simulink model "vekt_shim_PMSM"  (R2019b)
settings: Solver=ode4  StartTime=0.0  StopTime=10  FixedStep=1e-5  RelTol=1e-3
libraries: powerlib x4, simulink x3, powerlib_meascontrol x1
settings Model: Creator=Sozonov_AA  LastModifiedBy=Андрей
settings DataIOCC: SaveOutput=off  SaveTime=off
settings OptimizationCC: DefaultParameterBehavior=Inlined  InlineInvariantSignals=on  EnhancedBackFolding=on  PassReuseOutputArgsAs=Individual arguments  StateBitsets=on  DataBitsets=on  ZeroExternalMemoryAtStartup=off  ZeroInternalMemoryAtStartup=off  NoFixptDivByZeroProtection=on  EfficientFloat2IntCast=on  OptimizeBlockOrder=speed  DifferentSizesBufferReuse=on  EfficientTunableParamExpr=on
settings DebuggingCC: ParameterTunabilityLossMsg=error
settings SFSimCC: MATLABDynamicMemAlloc=off  CustomCodeUndefinedFunction=UseInterfaceOnly
settings RTWCC: SystemTargetFile=ert.tlc  TemplateMakefile=ert_default_tmf  GenerateReport=on  RTWVerbose=off  IncludeHyperlinkInReport=on  LaunchReport=on  GenerateTraceInfo=on  GenerateTraceReport=on  GenerateTraceReportSl=on  GenerateTraceReportSf=on  GenerateTraceReportEml=on
settings CodeAppCC: ForceParamTrailComments=on  IgnoreCustomStorageClasses=off  OperatorAnnotations=on  SimulinkDataObjDesc=on  SFDataObjDesc=on  CustomSymbolStrGlobalVar=rt$N$M  CustomSymbolStrType=$N$M  CustomSymbolStrFcn=$N$M$F  CustomSymbolStrMacro=$N$M  InsertBlockDesc=on
settings ERTTargetCC: TargetLangStandard=C99 (ISO)  GenerateSampleERTMain=on  IncludeMdlTerminateFcn=off  CombineSignalStateStructs=on  PurelyIntegerCode=on  SupportNonFinite=off  InlinedParameterPlacement=NonHierarchical  ERTCustomFileTemplate=example_file_process.tlc

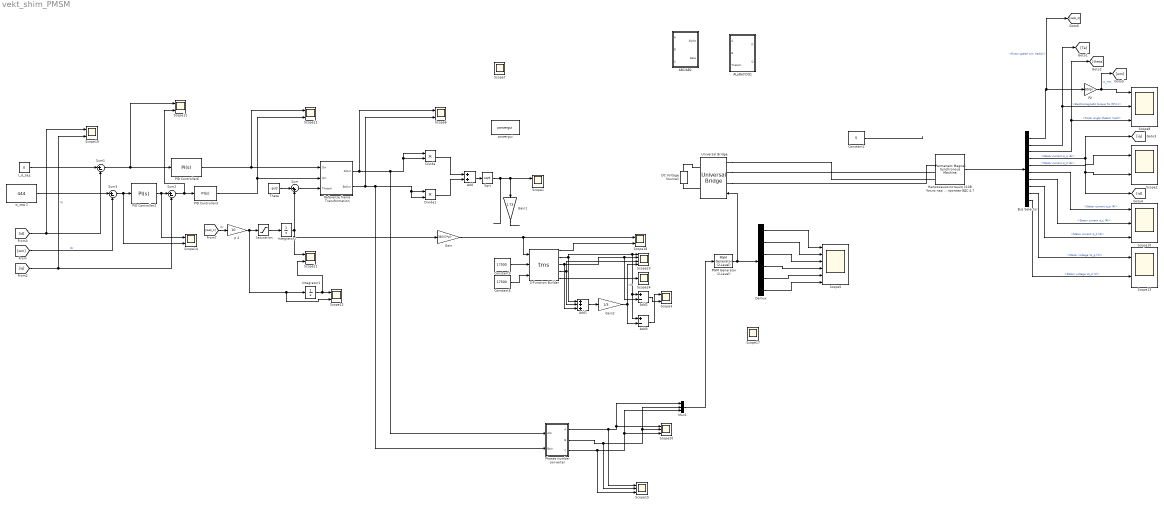
== system vekt_shim_PMSM ==
  "\tReferense frame Transformation" : Subsystem
  ABC/AB2 : Subsystem
  ALpBet\DQ1 : Subsystem
  Add : Sum
  Add1 : Sum  Inputs=+++
  Add2 : Sum  Inputs=+-
  Add3 : Sum  Inputs=+-
  Bus Selector : BusSelector  OutputSignals=Rotor speed wm (rad/s),Electromagnetic torque Te (N*m),Rotor angle thetam (rad),Stator current is_q (A),Stator current is_d (A),Stator current is_a (A),Stator current is_c (A),Stator current is_b (A),Stator voltage Vs_q (V),Stator voltage Vs_d (V)
  Constant2 : Constant  Value=5
  Constant3 : Constant  Value=17500
  Constant5 : Constant  Value=17500
  DC Voltage Source1 : powerlib/Electrical Sources/DC Voltage Source  Amplitude=310  Measurements=None
      settings: SourceProductName=Simscape Electrical
  Demux : Demux  Outputs=6
  Divide : Product  Inputs=**
  Divide1 : Product  Inputs=**
  Gain : Gain  Gain=360/(2*pi)
  Gain1 : Gain  Gain=1.73
  Gain2 : Gain  Gain=1/3
  I_d_зад : Constant  Value=0
  Integrator1 : Integrator  UpperSaturationLimit=2*pi  LowerSaturationLimit=0  WrappedStateUpperValue=2*pi  WrappedStateLowerValue=0  ZeroCross=off
  Integrator2 : Integrator  UpperSaturationLimit=2*pi  LowerSaturationLimit=0  WrapState=on  WrappedStateUpperValue=2*pi  WrappedStateLowerValue=0  ZeroCross=off
  Mux1 : Mux  Inputs=3
  P2 : Gain  Gain=30/pi
  PID Controller2 : simulink/Continuous/PID Controller  Controller=PI  Form=Ideal  TimeDomain=Continuous-time  SampleTime=-1  IntegratorMethod=Forward Euler  FilterMethod=Forward Euler  ControllerParametersSource=internal  P=16/444  I=(16/444)*150  D=0  UseFilter=on  N=100  TunerSelectOption=Transfer Function Based (PID Tuner App)  InitialConditionSource=internal  InitialConditionForIntegrator=0  InitialConditionForFilter=0  DifferentiatorICPrevScaledInput=0  ExternalReset=none  TrackingMode=off  Kt=1  LimitOutput=on  UpperSaturationLimit=1000  LowerSaturationLimit=-1000  LinearizeAsGain=on  AntiWindupMode=none  Kb=1  POutMin=[]  POutMax=[]  IOutMin=[]  IOutMax=[]  DOutMin=[]  DOutMax=[]  NOutMin=[]  NOutMax=[]  SumOutMin=[]  SumOutMax=[]  SaturationOutMin=[]  SaturationOutMax=[]  PParamMin=[]  PParamMax=[]  IParamMin=[]  IParamMax=[]  DParamMin=[]  DParamMax=[]  NParamMin=[]  NParamMax=[]  KbParamMin=[]  KbParamMax=[]  KtParamMin=[]  KtParamMax=[]  KbOutMin=[]  KbOutMax=[]  KtOutMin=[]  KtOutMax=[]  IntegratorOutMin=[]  IntegratorOutMax=[]  FilterOutMin=[]  FilterOutMax=[]  SumI1OutMin=[]  SumI1OutMax=[]  SumI2OutMin=[]  SumI2OutMax=[]  SumI3OutMin=[]  SumI3OutMax=[]  SumI4OutMin=[]  SumI4OutMax=[]  SumDOutMin=[]  SumDOutMax=[]  DifferentiatorOutMin=[]  DifferentiatorOutMax=[]  FilterDiffOutCoefMin=[]  FilterDiffOutCoefMax=[]  ReciprocalOutMin=[]  ReciprocalOutMax=[]  SumDenOutMin=[]  SumDenOutMax=[]  SumNumOutMin=[]  SumNumOutMax=[]  DivideOutMin=[]  DivideOutMax=[]  IntegratorContinuousStateAttributes=''  IntegratorStateMustResolveToSignalObject=off  IntegratorRTWStateStorageClass=Auto  FilterContinuousStateAttributes=''  FilterStateMustResolveToSignalObject=off  FilterRTWStateStorageClass=Auto  ParallelPVariant=Passthrough  IdealPVariant=InternalParameters  IVariant=InternalParameters  DVariant=Disabled  IntegratorVariant=Continuous  SatVariant=Enabled  AWVariant=Passthrough  PCopyVariant=Disabled  TRVariant=Disabled  FdbkBlocksVariant=Forward  IdealPFdbkVariant=Disabled  SatFdbkVariant=Disabled  DerivativeFilterVariant=Disabled  NVariant=Disabled  NCopyVariant=Disabled_SignalSpec  FilterICVariant=Disabled  IntegratorICVariant=InternalICs  ExternalResetVariant=Disabled  TRSumVariant=Passthrough  SumFdbkVariant=Disabled  SumVariant=Sum_PI
  PID Controller3 : simulink/Continuous/PID Controller  Controller=PI  Form=Ideal  TimeDomain=Continuous-time  SampleTime=-1  IntegratorMethod=Forward Euler  FilterMethod=Forward Euler  ControllerParametersSource=internal  P=220/0.5  I=(220/0.5)*4  D=0  UseFilter=on  N=100  TunerSelectOption=Transfer Function Based (PID Tuner App)  InitialConditionSource=internal  InitialConditionForIntegrator=0  InitialConditionForFilter=0  DifferentiatorICPrevScaledInput=0  ExternalReset=none  TrackingMode=off  Kt=1  LimitOutput=on  UpperSaturationLimit=1000  LowerSaturationLimit=-1000  LinearizeAsGain=on  AntiWindupMode=none  Kb=1  POutMin=[]  POutMax=[]  IOutMin=[]  IOutMax=[]  DOutMin=[]  DOutMax=[]  NOutMin=[]  NOutMax=[]  SumOutMin=[]  SumOutMax=[]  SaturationOutMin=[]  SaturationOutMax=[]  PParamMin=[]  PParamMax=[]  IParamMin=[]  IParamMax=[]  DParamMin=[]  DParamMax=[]  NParamMin=[]  NParamMax=[]  KbParamMin=[]  KbParamMax=[]  KtParamMin=[]  KtParamMax=[]  KbOutMin=[]  KbOutMax=[]  KtOutMin=[]  KtOutMax=[]  IntegratorOutMin=[]  IntegratorOutMax=[]  FilterOutMin=[]  FilterOutMax=[]  SumI1OutMin=[]  SumI1OutMax=[]  SumI2OutMin=[]  SumI2OutMax=[]  SumI3OutMin=[]  SumI3OutMax=[]  SumI4OutMin=[]  SumI4OutMax=[]  SumDOutMin=[]  SumDOutMax=[]  DifferentiatorOutMin=[]  DifferentiatorOutMax=[]  FilterDiffOutCoefMin=[]  FilterDiffOutCoefMax=[]  ReciprocalOutMin=[]  ReciprocalOutMax=[]  SumDenOutMin=[]  SumDenOutMax=[]  SumNumOutMin=[]  SumNumOutMax=[]  DivideOutMin=[]  DivideOutMax=[]  IntegratorContinuousStateAttributes=''  IntegratorStateMustResolveToSignalObject=off  IntegratorRTWStateStorageClass=Auto  FilterContinuousStateAttributes=''  FilterStateMustResolveToSignalObject=off  FilterRTWStateStorageClass=Auto  ParallelPVariant=Passthrough  IdealPVariant=InternalParameters  IVariant=InternalParameters  DVariant=Disabled  IntegratorVariant=Continuous  SatVariant=Enabled  AWVariant=Passthrough  PCopyVariant=Disabled  TRVariant=Disabled  FdbkBlocksVariant=Forward  IdealPFdbkVariant=Disabled  SatFdbkVariant=Disabled  DerivativeFilterVariant=Disabled  NVariant=Disabled  NCopyVariant=Disabled_SignalSpec  FilterICVariant=Disabled  IntegratorICVariant=InternalICs  ExternalResetVariant=Disabled  TRSumVariant=Passthrough  SumFdbkVariant=Disabled  SumVariant=Sum_PI
  PID Controller6 : simulink/Continuous/PID Controller  Controller=PI  Form=Ideal  TimeDomain=Continuous-time  SampleTime=-1  IntegratorMethod=Forward Euler  FilterMethod=Forward Euler  ControllerParametersSource=internal  P=220/20  I=(220/20)*35  D=0  UseFilter=on  N=100  TunerSelectOption=Transfer Function Based (PID Tuner App)  InitialConditionSource=internal  InitialConditionForIntegrator=0  InitialConditionForFilter=0  DifferentiatorICPrevScaledInput=0  ExternalReset=none  TrackingMode=off  Kt=1  LimitOutput=on  UpperSaturationLimit=1000  LowerSaturationLimit=-1000  LinearizeAsGain=on  AntiWindupMode=none  Kb=1  POutMin=[]  POutMax=[]  IOutMin=[]  IOutMax=[]  DOutMin=[]  DOutMax=[]  NOutMin=[]  NOutMax=[]  SumOutMin=[]  SumOutMax=[]  SaturationOutMin=[]  SaturationOutMax=[]  PParamMin=[]  PParamMax=[]  IParamMin=[]  IParamMax=[]  DParamMin=[]  DParamMax=[]  NParamMin=[]  NParamMax=[]  KbParamMin=[]  KbParamMax=[]  KtParamMin=[]  KtParamMax=[]  KbOutMin=[]  KbOutMax=[]  KtOutMin=[]  KtOutMax=[]  IntegratorOutMin=[]  IntegratorOutMax=[]  FilterOutMin=[]  FilterOutMax=[]  SumI1OutMin=[]  SumI1OutMax=[]  SumI2OutMin=[]  SumI2OutMax=[]  SumI3OutMin=[]  SumI3OutMax=[]  SumI4OutMin=[]  SumI4OutMax=[]  SumDOutMin=[]  SumDOutMax=[]  DifferentiatorOutMin=[]  DifferentiatorOutMax=[]  FilterDiffOutCoefMin=[]  FilterDiffOutCoefMax=[]  ReciprocalOutMin=[]  ReciprocalOutMax=[]  SumDenOutMin=[]  SumDenOutMax=[]  SumNumOutMin=[]  SumNumOutMax=[]  DivideOutMin=[]  DivideOutMax=[]  IntegratorContinuousStateAttributes=''  IntegratorStateMustResolveToSignalObject=off  IntegratorRTWStateStorageClass=Auto  FilterContinuousStateAttributes=''  FilterStateMustResolveToSignalObject=off  FilterRTWStateStorageClass=Auto  ParallelPVariant=Passthrough  IdealPVariant=InternalParameters  IVariant=InternalParameters  DVariant=Disabled  IntegratorVariant=Continuous  SatVariant=Enabled  AWVariant=Passthrough  PCopyVariant=Disabled  TRVariant=Disabled  FdbkBlocksVariant=Forward  IdealPFdbkVariant=Disabled  SatFdbkVariant=Disabled  DerivativeFilterVariant=Disabled  NVariant=Disabled  NCopyVariant=Disabled_SignalSpec  FilterICVariant=Disabled  IntegratorICVariant=InternalICs  ExternalResetVariant=Disabled  TRSumVariant=Passthrough  SumFdbkVariant=Disabled  SumVariant=Sum_PI
  PWM Generator (2-Level) : powerlib_meascontrol/Pulse & Signal Generators/PWM Generator (2-Level)  ModulatorType=Three-phase bridge (6 pulses)  ModulatorMode=Unsynchronized  Fc=1000  Pc=90  nF=27  MinMax="[ 0  1 ]"  SamplingTechnique=Natural  ModulatingSignals=off  m=0.8  Freq=60  Phase=0  Ts=0  ShowCarrierOutport=off
  Phases number converter : Subsystem
  S-Function Builder : S-Function  InitFcn=try, set_param(gcb,'FunctionName','tms'), end  FunctionName=tms  SFunctionModules=tms_wrapper svpwm  SFunctionDeploymentMode=off  EnableBusSupport=off  mask(S-Function Builder){}
      mask help: Simulink:masks:SFunctionBuilder_MD
      mask init:
      | val = [[.9  0.75 0.75 1 1 .9 .9 1]',[1 1 0.75 0.75 .9 .9 1 .9]'];try , sys = get_param(gcb,'SfunBuilderFcnName');if isempty(sys), sys = get_param(gcb,'FunctionName'); end,catch, sys = get_param(gcb,'FunctionName'); end
      settings: CopyFcn=set_param(gcbh,'LinkStatus','none')  PreSaveFcn=try, set_param(gcb,'FunctionName','tms'), end  OpenFcn=sfunctionwizard(gcbh)
      mask Display:
      | plot(val(:,1),val(:,2))
      | disp(sys)
      | port_label('input',1,'wt_i')
      | port_label('input',2,'ud_i')
      | port_label('input',3,'us_a_i')
      | port_label('output',1,'betta_o')
      | port_label('output',2,'Ta_o')
      | port_label('output',3,'Tb_o')
      | port_label('output',4,'Tc_o')
      | port_label('output',5,'Us_o')
  Saturation : Saturate  UpperLimit=inf  LowerLimit=0
  Scope{1..3,6,11..14,18..19,21..22} (12 alike) : Scope  NumInputPorts=2
  Scope{8,10,15,20} (4 alike) : Scope  NumInputPorts=3
  Scope17 : Scope  NumInputPorts=4
  Scope23 : Scope  NumInputPorts=4
  Scope24 : Scope
  Scope5 : Scope  NumInputPorts=6
  Scope7 : Scope
  Sqrt : Sqrt  SaturateOnIntegerOverflow=on
  Sum : Sum  Inputs=|++
  Sum1 : Sum  Inputs=|+-
  Sum2 : Sum  Inputs=|+-
  Sum3 : Sum  Inputs=|+-
  Theta : Constant  Value=-pi/2
  Universal Bridge : powerlib/Power Electronics/Universal Bridge  Arms=3  SnubberResistance=1e5  SnubberCapacitance=inf  Device=IGBT / Diodes  Ron=1e-3  Lon=0  ForwardVoltages="[  0  0  ]"  ForwardVoltage=0  GTOparameters=[ 10e-6 , 20e-6 ]  IGBTparameters=[ 1e-6 , 2e-6 ]  Measurements=None  Measurements_2=None  converterType=Rectifier
      settings: SourceProductName=Simscape Electrical
  p 2 : Gain  Gain=10
  powergui : powerlib/powergui  Priority=1  SimulationMode=Discrete  SampleTime=2e-5  frequency=60  Iterations=50  frequencyindice=0  Pbase=100e6  ErrMax=1e-4  UnitsV=kV  UnitsW=MW  buscounter=0  FunctionMessages=off  echomessages=off  EnableUseOfTLC=off  CurrentSourceSwitches=off  DisableSnubberDevices=off  DisableRonSwitches=off  DisableVfSwitches=off  DisplayEquations=off  AutomaticDiscreteSolvers=off  SolverType=Tustin/Backward Euler (TBE)  Interpol=off  ExternalGateDelay=off  methode=off  Ts=100  x0status=blocks  SPID=on  SwTol=0  HookPort=off  NonlinearTolerance=0  nMaxIteration=15  ContinueOnMaxIteration=off  RestoreLinks=warning  ResistiveCurrentMeasurement=off  Frange=[0:2:500]  Ylog=off  Xlog=on  ShowGrid=off  save=off  variable=ZData  structure=0  ZoomFFT=off  StartTime=0.0  cycles=1  DisplayStyle=1  fundamental=60  FreqAxis=off  MaxFrequency=1000  frequencyindicesteady=1  RmsSteady=1  display=off
      settings: SourceProductName=Simscape Electrical
  w_зад 2 : Constant  Value=444
  "Напряжения питания 310В. Число пар полюсов 10. Момент инерции ротора 0,003 кг/м2 . Длит. момент возд. охл. 19,5 Нм. Момент трения в подшипниках 1 Нм. Зубцовый момент 1 Нм. Максимальная скорость при Ma 444 об/мин. Скорость холостого хода при Mb 533 об/мин. Длит. ток с возд. охл. 3,4 А. Ток ХХ при Mb и Nb 0,7 А. КПД при Ma и Us 84,1%. Электрическое сопротивление при 20 град. Цельсия 5,92 Ом. Индуктивность 39,8 мГн. Коэффициент момента 5,7. Коэффициент противо-ЭДС 4,7 " : powerlib/Machines/Permanent Magnet Synchronous Machine  NbPhases=3  FluxDistribution=Sinusoidal  RotorType=Round  MechanicalLoad=Torque Tm  PresetModel=No  ShowDetailedParameters=on  MeasurementBus=off  Resistance=5.92  Inductance=8.5e-3  dqInductances=[8.5e-3,8.5e-3]  La=(39.8e-3)/2  MachineConstant=Voltage Constant (V_peak L-L / krpm)  Flux=0.38  VoltageCst=689.2438  TorqueCst=5.7  Flat=120  Mechanical=[0.003 0 10 0]  PolePairs=4  InitialConditions=[0,0, 0,0]  InitialConditions5ph=[0 0 0 0 0 0]  RefAngle=90 degrees behind phase A axis (modified Park)  IterativeDiscreteModel=Trapezoidal non iterative  TsBlock=-1  TsPowergui=0
  wires:
  Gain/1 -> S-Function Builder/1, Scope18/1
  "\tReferense frame Transformation"/1(AlOut) -> Scope6/1, Phases number converter/1(AlIn), Divide/1, Divide/2
  Add/1 -> Sqrt/1
  Divide/1 -> Add/1
  Divide1/1 -> Add/2
  Sqrt/1 -> Scope1/1, Gain1/1
  Demux/1 -> Scope5/1
  Demux/2 -> Scope5/2
  Demux/3 -> Scope5/3
  Demux/4 -> Scope5/4
  Demux/5 -> Scope5/5
  Demux/6 -> Scope5/6
  PWM Generator (2-Level)/1 -> Universal Bridge/1, Demux/1
  "Напряжения питания 310В. Число пар полюсов 10. Момент инерции ротора 0,003 кг/м2 . Длит. момент возд. охл. 19,5 Нм. Момент трения в подшипниках 1 Нм. Зубцовый момент 1 Нм. Максимальная скорость при Ma 444 об/мин. Скорость холостого хода при Mb 533 об/мин. Длит. ток с возд. охл. 3,4 А. Ток ХХ при Mb и Nb 0,7 А. КПД при Ma и Us 84,1%. Электрическое сопротивление при 20 град. Цельсия 5,92 Ом. Индуктивность 39,8 мГн. Коэффициент момента 5,7. Коэффициент противо-ЭДС 4,7 "/1 -> Bus Selector/1
  [iq] -> Scope19/2, Sum2/2  "Iq"
  Bus Selector/1 -> [rads_1], P2/1  "<Rotor speed wm (rad/s)>"
  Bus Selector/2 -> [Te], Scope8/2  "<Electromagnetic torque Te (N*m)>"
  Bus Selector/4 -> Scope2/1, [iq]  "<Stator current is_q (A)>"
  Bus Selector/5 -> [id], Scope2/2  "<Stator current is_d (A)>"
  Bus Selector/6 -> Scope10/1  "<Stator current is_a (A)>"
  Bus Selector/7 -> Scope10/2  "<Stator current is_c (A)>"
  Bus Selector/8 -> Scope10/3  "<Stator current is_b (A)>"
  Bus Selector/3 -> [theta], Scope8/3  "<Rotor angle thetam (rad)>"
  "\tReferense frame Transformation"/2(BeOut) -> Scope6/2, Phases number converter/2(Bein), Divide1/2, Divide1/1
  w_зад 2/1 -> Sum3/1
  PID Controller2/1 -> Scope14/1, Sum2/1
  Sum2/1 -> Scope12/2, PID Controller3/1
  Sum3/1 -> Scope14/2, PID Controller2/1
  Sum1/1 -> PID Controller6/1, Scope12/1
  [id] -> Scope19/1, Sum1/2
  [wm] -> Sum3/2  "Nr"
  Theta/1 -> Sum/1
  Sum/1 -> "\tReferense frame Transformation"/3(ThetaIn)
  Phases number converter/1(A) -> Scope15/1, Scope20/1, Mux1/1
  Phases number converter/2(B) -> Scope15/2, Scope20/2, Mux1/2
  Phases number converter/3(C) -> Scope15/3, Scope20/3, Mux1/3
  P2/1 -> [wm], Scope8/1  "w_тек"
  Bus Selector/9 -> Scope13/1  "<Stator voltage Vs_q (V)>"
  Bus Selector/10 -> Scope13/2  "<Stator voltage Vs_d (V)>"
  Gain1/1 -> ?
  Mux1/1 -> PWM Generator (2-Level)/1
  PID Controller6/1 -> "\tReferense frame Transformation"/1(Din), Scope11/1
  PID Controller3/1 -> "\tReferense frame Transformation"/2(Qin), Scope11/2
  I_d_зад/1 -> Sum1/1
  Constant2/1 -> ?
  [rads_1] -> p 2/1  "Nr"
  Integrator2/1 -> Scope21/1, Gain/1, Sum/2
  Integrator1/1 -> Scope21/2, Scope22/1
  p 2/1 -> Saturation/1, Scope22/2, Integrator1/1
  Saturation/1 -> Integrator2/1
  Constant3/1 -> S-Function Builder/2
  Constant5/1 -> S-Function Builder/3
  S-Function Builder/1 -> Scope18/2
  S-Function Builder/2 -> Add1/1, Add3/1, Add2/1, Scope23/1
  S-Function Builder/3 -> Add1/3, Add2/2, Scope23/2
  S-Function Builder/4 -> Add1/2, Scope23/3
  S-Function Builder/5 -> Scope24/1
  Add1/1 -> Gain2/1
  Gain2/1 -> Add3/2, Scope23/4  "U0"
  Add2/1 -> Scope3/2
  Add3/1 -> Scope3/1
  connections:
  Universal Bridge/LConn1 -- "Напряжения питания 310В. Число пар полюсов 10. Момент инерции ротора 0,003 кг/м2 . Длит. момент возд. охл. 19,5 Нм. Момент трения в подшипниках 1 Нм. Зубцовый момент 1 Нм. Максимальная скорость при Ma 444 об/мин. Скорость холостого хода при Mb 533 об/мин. Длит. ток с возд. охл. 3,4 А. Ток ХХ при Mb и Nb 0,7 А. КПД при Ma и Us 84,1%. Электрическое сопротивление при 20 град. Цельсия 5,92 Ом. Индуктивность 39,8 мГн. Коэффициент момента 5,7. Коэффициент противо-ЭДС 4,7 "/LConn1
  Universal Bridge/LConn3 -- "Напряжения питания 310В. Число пар полюсов 10. Момент инерции ротора 0,003 кг/м2 . Длит. момент возд. охл. 19,5 Нм. Момент трения в подшипниках 1 Нм. Зубцовый момент 1 Нм. Максимальная скорость при Ma 444 об/мин. Скорость холостого хода при Mb 533 об/мин. Длит. ток с возд. охл. 3,4 А. Ток ХХ при Mb и Nb 0,7 А. КПД при Ma и Us 84,1%. Электрическое сопротивление при 20 град. Цельсия 5,92 Ом. Индуктивность 39,8 мГн. Коэффициент момента 5,7. Коэффициент противо-ЭДС 4,7 "/LConn3
  Universal Bridge/LConn2 -- "Напряжения питания 310В. Число пар полюсов 10. Момент инерции ротора 0,003 кг/м2 . Длит. момент возд. охл. 19,5 Нм. Момент трения в подшипниках 1 Нм. Зубцовый момент 1 Нм. Максимальная скорость при Ma 444 об/мин. Скорость холостого хода при Mb 533 об/мин. Длит. ток с возд. охл. 3,4 А. Ток ХХ при Mb и Nb 0,7 А. КПД при Ma и Us 84,1%. Электрическое сопротивление при 20 град. Цельсия 5,92 Ом. Индуктивность 39,8 мГн. Коэффициент момента 5,7. Коэффициент противо-ЭДС 4,7 "/LConn2
  DC Voltage Source1/RConn1 -- Universal Bridge/RConn1
  DC Voltage Source1/LConn1 -- Universal Bridge/RConn2

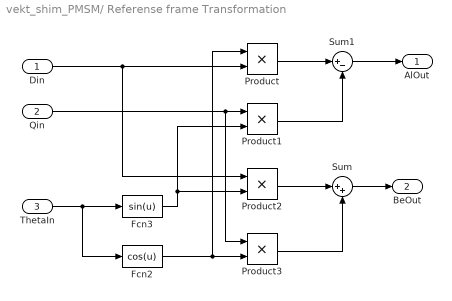
== system vekt_shim_PMSM/	Referense frame Transformation ==
  Din : Inport
  Qin : Inport  Port=2
  ThetaIn : Inport  Port=3
  Fcn2 : Fcn  Expr=cos(u)
  Fcn3 : Fcn  Expr=sin(u)
  Product{,1..3} (4 alike) : Product  RndMeth=Zero
  Sum : Sum  Inputs=|++
  Sum1 : Sum  Inputs=|+-
  AlOut : Outport  VectorParamsAs1DForOutWhenUnconnected=off
  BeOut : Outport  Port=2  VectorParamsAs1DForOutWhenUnconnected=off
  wires:
  ThetaIn/1 -> Fcn2/1, Fcn3/1
  Product/1 -> Sum1/1
  Product1/1 -> Sum1/2
  Sum1/1 -> AlOut/1
  Sum/1 -> BeOut/1
  Product2/1 -> Sum/1
  Product3/1 -> Sum/2
  Fcn2/1 -> Product/1, Product3/2
  Din/1 -> Product/2, Product2/1
  Qin/1 -> Product3/1, Product1/1
  Fcn3/1 -> Product1/2, Product2/2

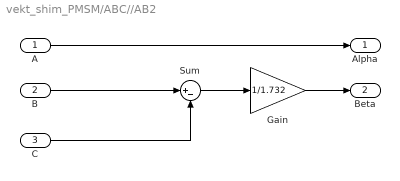
== system vekt_shim_PMSM/ABC//AB2 ==
  A : Inport
  B : Inport  Port=2
  C : Inport  Port=3
  Gain : Gain  Gain=1/1.732
  Sum : Sum  Inputs=|+-
  Alpha : Outport  VectorParamsAs1DForOutWhenUnconnected=off
  Beta : Outport  Port=2  VectorParamsAs1DForOutWhenUnconnected=off
  wires:
  Gain/1 -> Beta/1
  A/1 -> Alpha/1
  Sum/1 -> Gain/1
  C/1 -> Sum/2
  B/1 -> Sum/1

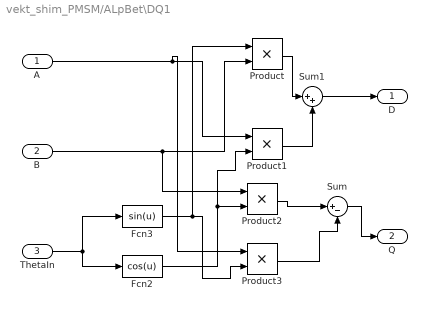
== system vekt_shim_PMSM/ALpBet\DQ1 ==
  A : Inport
  B : Inport  Port=2
  ThetaIn : Inport  Port=3
  Fcn2 : Fcn  Expr=cos(u)
  Fcn3 : Fcn  Expr=sin(u)
  Product{,1..3} (4 alike) : Product  RndMeth=Zero
  Sum : Sum  Inputs=|+-
  Sum1 : Sum  Inputs=|++
  D : Outport  VectorParamsAs1DForOutWhenUnconnected=off
  Q : Outport  Port=2  VectorParamsAs1DForOutWhenUnconnected=off
  wires:
  Product3/1 -> Sum/2
  Product2/1 -> Sum/1
  Sum/1 -> Q/1
  Sum1/1 -> D/1
  Product1/1 -> Sum1/2
  Product/1 -> Sum1/1
  A/1 -> Product3/1, Product1/1
  Fcn2/1 -> Product2/2, Product1/2
  Fcn3/1 -> Product3/2, Product/1
  B/1 -> Product2/1, Product/2
  ThetaIn/1 -> Fcn2/1, Fcn3/1

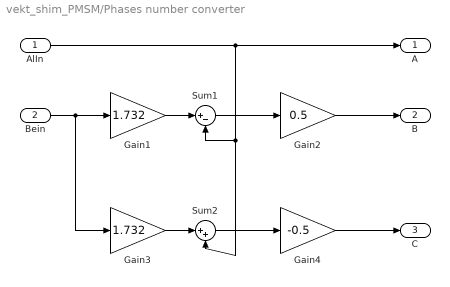
== system vekt_shim_PMSM/Phases number converter ==
  AlIn : Inport
  Bein : Inport  Port=2
  Gain1 : Gain  Gain=1.732
  Gain2 : Gain  Gain=0.5
  Gain3 : Gain  Gain=1.732
  Gain4 : Gain  Gain=-0.5
  Sum1 : Sum  Inputs=|+-
  Sum2 : Sum  Inputs=|++
  A : Outport  VectorParamsAs1DForOutWhenUnconnected=off
  B : Outport  Port=2  VectorParamsAs1DForOutWhenUnconnected=off
  C : Outport  Port=3  VectorParamsAs1DForOutWhenUnconnected=off
  wires:
  AlIn/1 -> A/1, Sum1/2, Sum2/2
  Bein/1 -> Gain1/1, Gain3/1
  Gain1/1 -> Sum1/1
  Sum1/1 -> Gain2/1
  Gain2/1 -> B/1
  Gain3/1 -> Sum2/1
  Sum2/1 -> Gain4/1
  Gain4/1 -> C/1
